simulink model "test"  (R2016a)
settings: Solver=FixedStepDiscrete  StartTime=0.0  StopTime=10.0  RelTol=1e-3
settings Model: ExtModeTrigDuration=2  Creator=shohei  LastModifiedBy=shohei
settings OptimizationCC: OptimizeModelRefInitCode=on  LifeSpan=1  MaxStackSize=64
settings HardwareCC: ProdBitPerInt=16  ProdBitPerPointer=16  ProdLargestAtomicFloat=None  ProdWordSize=8  ProdHWDeviceType=Atmel->AVR
settings RTWCC: SystemTargetFile=ert.tlc  HardwareBoard=Arduino Uno  TemplateMakefile=ert_default_tmf  GenerateReport=on  Toolchain=Arduino AVR v1.6.1  BuildConfiguration=Faster Runs  IncludeHyperlinkInReport=on  LaunchReport=on  GenerateTraceInfo=on  GenerateTraceReport=on  GenerateTraceReportSl=on  GenerateTraceReportSf=on  GenerateTraceReportEml=on
settings CodeAppCC: ForceParamTrailComments=on  IgnoreCustomStorageClasses=off  OperatorAnnotations=on  SimulinkDataObjDesc=on  SFDataObjDesc=on  MATLABFcnDesc=on  MangleLength=10  InsertBlockDesc=on  MATLABSourceComments=on
settings ERTTargetCC: SupportContinuousTime=on  SupportVariableSizeSignals=on  ExtMode=on  ExtModeTransport=3  ExtModeMexFile=ext_serial_win32_comm_rtt  ExtModeMexArgs=0 '/dev/cu.usbmodem1421' 115200

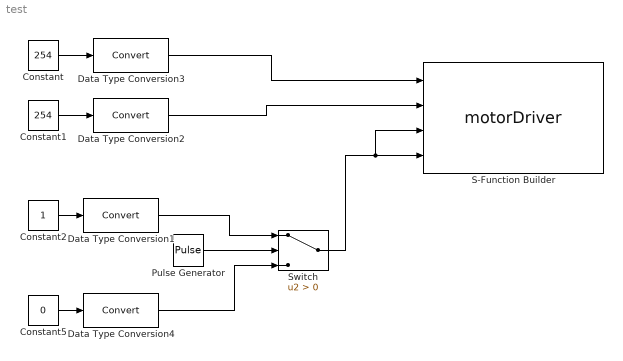
== system test ==
  Constant : Constant  Value=254
  Constant1 : Constant  Value=254
  Constant2 : Constant
  Constant5 : Constant  Value=0
  Data Type Conversion{1..4} (4 alike) : DataTypeConversion
  Pulse Generator : DiscretePulseGenerator  PulseType=Time based  Period=4  PulseWidth=50
  S-Function Builder : S-Function  InitFcn=try, set_param(gcb,'FunctionName','motorDriver'), end  FunctionName=motorDriver  SFunctionModules=motorDriver_wrapper  SFunctionDeploymentMode=off  EnableBusSupport=off  mask(S-Function Builder){}
      mask help: Simulink:masks:SFunctionBuilder_MD
      mask init:
      | val = [[.9  0.75 0.75 1 1 .9 .9 1]',[1 1 0.75 0.75 .9 .9 1 .9]'];try , sys = get_param(gcb,'SfunBuilderFcnName');if isempty(sys), sys = get_param(gcb,'FunctionName'); end,catch, sys = get_param(gcb,'FunctionName'); end
      settings: CopyFcn=set_param(gcbh,'LinkStatus','none')  PreSaveFcn=try, set_param(gcb,'FunctionName','motorDriver'), end  OpenFcn=sfunctionwizard(gcbh)
      mask Display: plot(val(:,1),val(:,2)),disp(sys), port_label('input',1,'speed1'), port_label('input',2,'speed2'), port_label('input',3,'direction1'), port_label('input',4,'direction2')
  Switch : Switch  Criteria=u2 > Threshold
  wires:
  Constant/1 -> Data Type Conversion3/1
  Constant1/1 -> Data Type Conversion2/1
  Constant2/1 -> Data Type Conversion1/1
  Data Type Conversion3/1 -> S-Function Builder/1
  Data Type Conversion2/1 -> S-Function Builder/2
  Data Type Conversion1/1 -> Switch/1
  Pulse Generator/1 -> Switch/2
  Data Type Conversion4/1 -> Switch/3
  Constant5/1 -> Data Type Conversion4/1
  Switch/1 -> S-Function Builder/3, S-Function Builder/4
